simulink model "SimulinkModelEs2"  (R2023a)
settings: Solver=VariableStepAuto  StartTime=0.0  StopTime=100.0  RelTol=1e-3
undefined symbols (not defined in the file or in its folder): fdesignblkfcn, gcbh
libraries: dspfdesign x4, vrlib x1
settings Model: Creator=pisy1  LastModifiedBy=pisy1

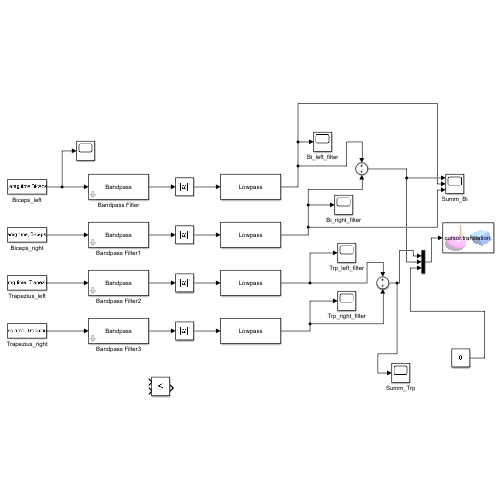
[thumbnail: Simulink's stored preview of the top-level diagram]
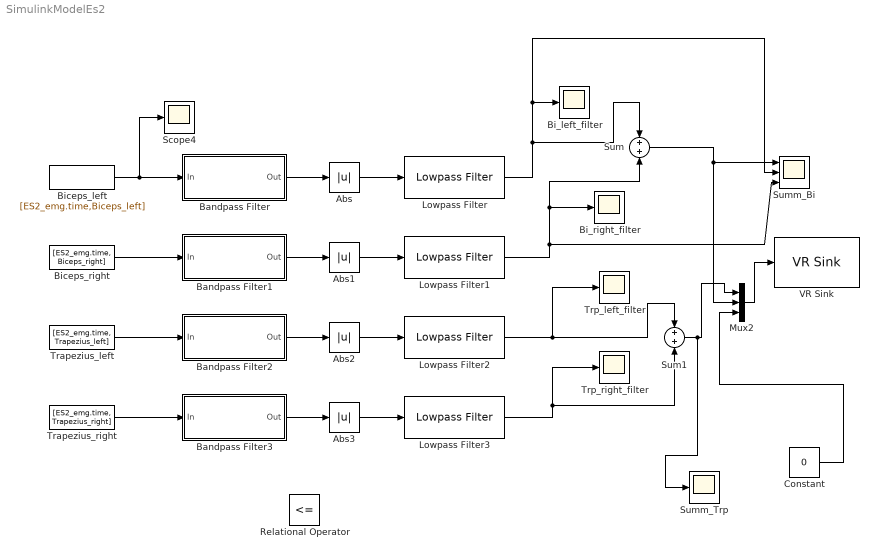
== system SimulinkModelEs2 ==
  Abs{,1..3} (4 alike) : Abs  SaturateOnIntegerOverflow=off
  Bandpass Filter : Subsystem  DialogController=fdesignblkfcn  InitFcn=fdesignblkfcn(gcbh, {'InitFcn'});  mask(Bandpass Filter){}
      mask help: dsp:DSPFilterDesignBlockDialog:BandpassFdesign_MaskDesc
      settings: CopyFcn=fdesignblkfcn(gcbh, {'CopyFcn'});
      mask Help: helpview(mapfilelocation('dsp'), 'dspbandpassfilter');
      mask Display: disp('Bandpass');
  Bandpass Filter1 : Subsystem  DialogController=fdesignblkfcn  InitFcn=fdesignblkfcn(gcbh, {'InitFcn'});  mask(Bandpass Filter){}
      mask help: dsp:DSPFilterDesignBlockDialog:BandpassFdesign_MaskDesc
      settings: CopyFcn=fdesignblkfcn(gcbh, {'CopyFcn'});
      mask Help: helpview(mapfilelocation('dsp'), 'dspbandpassfilter');
      mask Display: disp('Bandpass');
  Bandpass Filter2 : Subsystem  DialogController=fdesignblkfcn  InitFcn=fdesignblkfcn(gcbh, {'InitFcn'});  mask(Bandpass Filter){}
      mask help: dsp:DSPFilterDesignBlockDialog:BandpassFdesign_MaskDesc
      settings: CopyFcn=fdesignblkfcn(gcbh, {'CopyFcn'});
      mask Help: helpview(mapfilelocation('dsp'), 'dspbandpassfilter');
      mask Display: disp('Bandpass');
  Bandpass Filter3 : Subsystem  DialogController=fdesignblkfcn  InitFcn=fdesignblkfcn(gcbh, {'InitFcn'});  mask(Bandpass Filter){}
      mask help: dsp:DSPFilterDesignBlockDialog:BandpassFdesign_MaskDesc
      settings: CopyFcn=fdesignblkfcn(gcbh, {'CopyFcn'});
      mask Help: helpview(mapfilelocation('dsp'), 'dspbandpassfilter');
      mask Display: disp('Bandpass');
  Bi_left_filter : Scope
  Bi_right_filter : Scope
  Biceps_left : FromWorkspace  VariableName=[ES2_emg.time,Biceps_left]  SampleTime=1/1000
  Biceps_right : FromWorkspace  VariableName=[ES2_emg.time, Biceps_right]  SampleTime=1/1000
  Constant : Constant  Value=0
  Lowpass Filter{,1..3} (4 alike) : dspfdesign/Lowpass Filter  FilterType=FIR  DesignForMinimumOrder=on  FilterOrder=50  PassbandFrequency=3  StopbandFrequency=6  PassbandRipple=0.1  StopbandAttenuation=80  SampleRateMode=Specify on dialog  SampleRate=1000  SimulateUsing=Interpreted execution  roundingMode=Floor  coeffsDataTypeStr=fixdt(1,16)
  Mux2 : Mux  Inputs=3
  Relational Operator : RelationalOperator  Operator=<=  OutDataTypeStr=boolean  RndMeth=Simplest  InputSameDT=off
  Scope4 : Scope
  Sum : Sum  Inputs=+|+
  Sum1 : Sum  Inputs=+|+
  Summ_Bi : Scope  NumInputPorts=3
  Summ_Trp : Scope
  "Trapezius_left " : FromWorkspace  VariableName=[ES2_emg.time, Trapezius_left]  SampleTime=1/1000
  Trapezius_right : FromWorkspace  VariableName=[ES2_emg.time, Trapezius_right]  SampleTime=1/1000
  Trp_left_filter : Scope
  Trp_right_filter : Scope
  VR Sink : vrlib/VR Sink  InstantiateOnLoad=on  SampleTime=0.01  ViewEnable=on  RemoteChange=off  RemoteView=off  FieldsWritten=cursor.translation.3.1.1.double  WorldFileName=8_palline_color.wrl  AutoView=off  VideoDimensions=[]  AllowVariableSize=off  FigureProperties="{'Position', 'Name', 'Viewpoint', 'CameraBound', 'CameraDirection', 'CameraPosition', 'CameraUpVector', 'ZoomFactor', 'Antialiasing', 'Headlight', 'Lighting', 'NavPanel', 'Sound', 'StatusBar', 'Stereo3D', 'Stereo3DCameraOffset', 'Stereo3DHIT', 'ToolBar', 'Textures', 'Transparency', 'Triad', 'Wireframe', 'NavZones', 'NavMode', 'NavSpeed', 'CaptureFileFormat', 'CaptureFileName', 'Record2DCompressMethod', 'Record2DCompressQuality', 'Record2D', 'Record2DFileName', 'Record2DFPS'; [5.0000000000000000e+00   9.2000000000000000e+01   5.7600000000000000e+02   3.5000000000000000e+02], '', '_untitled_1', 'on', [0.0000000000000000e+00   0.0000000000000000e+00  -1.0000000000000000e+00], [0.0000000000000000e+00   0.0000000000000000e+00   3.0000000000000000e+00], [0.0000000000000000e+00   1.0000000000000000e+00   0.0000000000000000e+00], [1.0000000000000000e+00], 'on', 'on', 'on', 'halfbar', 'on', 'on', 'off', [1.0000000149011612e-01], [0.0000000000000000e+00], 'on', 'on', 'on', 'none', 'off', 'off', 'fly', 'normal', 'tif', '%f_anim_%n.tif', 'auto', [7.5000000000000000e+01], 'off', '%f_anim_%n.avi', 'auto'}"
  wires:
  Biceps_left/1 -> Scope4/1, Bandpass Filter/1(In)
  Bandpass Filter/1(Out) -> Abs/1
  Abs/1 -> Lowpass Filter/1
  Abs1/1 -> Lowpass Filter1/1
  Bandpass Filter1/1(Out) -> Abs1/1
  Biceps_right/1 -> Bandpass Filter1/1(In)
  Abs2/1 -> Lowpass Filter2/1
  Bandpass Filter2/1(Out) -> Abs2/1
  "Trapezius_left "/1 -> Bandpass Filter2/1(In)
  Trapezius_right/1 -> Bandpass Filter3/1(In)
  Abs3/1 -> Lowpass Filter3/1
  Bandpass Filter3/1(Out) -> Abs3/1
  Lowpass Filter3/1 -> Sum1/2, Trp_right_filter/1
  Lowpass Filter2/1 -> Trp_left_filter/1, Sum1/1
  Lowpass Filter1/1 -> Sum/2, Bi_right_filter/1, Summ_Bi/3
  Constant/1 -> Mux2/3
  Mux2/1 -> VR Sink/1
  Sum1/1 -> Summ_Trp/1, Mux2/1
  Lowpass Filter/1 -> Summ_Bi/2, Bi_left_filter/1, Sum/1
  Sum/1 -> Mux2/2, Summ_Bi/1

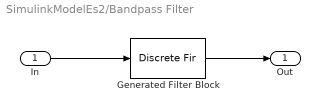
== system SimulinkModelEs2/Bandpass Filter ==
  In : Inport
  Generated Filter Block : DiscreteFir  Tag=BlockMethodSubSystem  Coefficients=[-9.3686702536914806e-06 3.12112809195631884e-05 -4.11531312163778077e-05 3.46959070674858323e-05 -6.95996272654917275e-05 2.25266942632591132e-05 -8.52586640162886797e-05 -1.01275601966525663e-05 -8.19699192663462454e-05 -6.15603887343607549e-05 -5.9928103484218156e-05 -0.000121773920488128754 -2.66693180046293347e-05 -0.000173582148305583721 4.85841196753850187e-06 -0.000196865446555221654 2.09241600116936787e-05 -0.000175070409473414502 1.29594738164580086e-05 -0.00010196560853616344 -1.73899410626521334e-05 1.38497153315267659e-05 -5.64059785452916983e-05 0.000148823711527270122 -8.11137804989736459e-05 0.000269600500847764297 -6.66819945948280264e-05 0.000342503652881703965 3.52069345312515154e-06 0.000344637780110196995 0.00012858070014359381 0.000272834014614537618 0.000285186521797195773 0.000146850926915565155 0.000430093252576786299 4.80147099397023455e-06 0.000510533795609378915 -0.000108659463339479432 0.000480381118947913633 -0.00015808597112364732 0.00031736039761362674 -0.000131661302689836559 3.54013407976428411e-05 -4.87012688565813937e-05 -0.000313041458963056755 4.36426183964740697e-05 -0.00064715606616753366 8.49659330390565632e-05 -0.000878874215356443373 2.38674809802090746e-05 -0.000939300192907026733 -0.000159137006239270498 -0.000802214987435227755 -0.000436425707633868653 -0.000496300153583344693 -0.000732724227282986296 -0.00010054958859877141 -0.00094194330334548609 0.000277523992628194436 -0.000958361368208270319 0.000535344128008414838 -0.000713561015643481011 0.000610103531338323461 -0.000207204782800491044 0.0005029728868787669 0.000479885492686017517 0.000282971816365619878 0.00119743844849929618 6.67763691850669971e-05 0.00176183555280003839 -2.12223470167560569e-05 0.00200788377478970615 0.000103228849646334322 0.00184114661190210136 0.000444622959401494813 0.00127370296145404597 0.000911631333604090194 0.00042976760914902062 0.00133366080069442696 -0.000483818369086393022 0.00150886983424911004 -0.00123599533659225617 0.00127138209007837677 -0.0016422211688103404 0.000557171809006548895 -0.00162513552744896839 -0.000554153422263470546 -0.00124390348382837166 -0.00183920406010100218 -0.000679478097852773263 -0.00297800611694112958 -0.000176737254097106202 -0.0036391164319655952 4.07217243879186256e-05 -0.00357950507876916542 -0.000143667762747536943 -0.0027285210290573284 -0.000682996094840989938 -0.00122710494485526902 -0.00136279543137825189 0.000594984672058177454 -0.00185700203672085201 0.00230266556106554403 -0.00183196437326688718 0.00347853357357814138 -0.00106869689246484384 0.00384924642170408025 0.000436157962248056197 0.00337472332535589245 0.00242774919190852931 0.00226811716984190578 0.00443079990486730003 0.000934428117831991511 0.00586565518688552268 -0.000158568641836894143 0.00621447784239509155 -0.00063968506314412716 0.00518988902168367443 -0.000372975212782562294 0.00285228027553475648 0.000473327518819695217 -0.000367190639521300702 0.00145817426323067989 -0.00375510870797710842 0.00199954564111136943 -0.00649909557305363567 0.00157338850405358815 -0.00791733371223253199 -7.98017159677944681e-05 -0.00766646088654352603 -0.00280949633821852727 -0.00586057658312818218 -0.00602733517521191614 -0.00305626313527977179 -0.00882178250879370185 -9.71425214211978983e-05 -0.0101967846478441017 0.0021442428271443801 -0.0093740351268534923 0.00305308159625901051 -0.00607123588018848061 0.0024971374225030039 -0.000666271859919423284 0.000910364244497557169 0.00581734844136641907 -0.000807046086893129476 0.0119203579027810664 -0.00156048754052804089 0.0161114922324175069 -0.00043720534318062381 0.0172127205975105453 0.00292079817401565914 0.0147655911445284671 0.00806627663117549971 0.0092239105285639323 0.013713884927239137 0.00189815567585120454 0.0179653836624237111 -0.00535739543202795598 0.0187613939058622961 -0.0106502874184987474 0.014459080896858505 -0.0126233469724383804 0.00438953523919432403 -0.0109426370703246453 -0.0107580013276019799 -0.00656125274562321687 ...(+4671 chars)]  InputProcessing=Columns as channels (frame based)
  Out : Outport  VectorParamsAs1DForOutWhenUnconnected=off
  wires:
  In/1 -> Generated Filter Block/1
  Generated Filter Block/1 -> Out/1

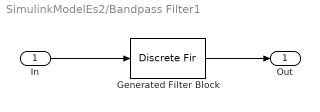
== system SimulinkModelEs2/Bandpass Filter1 ==
  In : Inport
  Generated Filter Block : DiscreteFir  Tag=BlockMethodSubSystem  Coefficients=[-9.3686702536914806e-06 3.12112809195631884e-05 -4.11531312163778077e-05 3.46959070674858323e-05 -6.95996272654917275e-05 2.25266942632591132e-05 -8.52586640162886797e-05 -1.01275601966525663e-05 -8.19699192663462454e-05 -6.15603887343607549e-05 -5.9928103484218156e-05 -0.000121773920488128754 -2.66693180046293347e-05 -0.000173582148305583721 4.85841196753850187e-06 -0.000196865446555221654 2.09241600116936787e-05 -0.000175070409473414502 1.29594738164580086e-05 -0.00010196560853616344 -1.73899410626521334e-05 1.38497153315267659e-05 -5.64059785452916983e-05 0.000148823711527270122 -8.11137804989736459e-05 0.000269600500847764297 -6.66819945948280264e-05 0.000342503652881703965 3.52069345312515154e-06 0.000344637780110196995 0.00012858070014359381 0.000272834014614537618 0.000285186521797195773 0.000146850926915565155 0.000430093252576786299 4.80147099397023455e-06 0.000510533795609378915 -0.000108659463339479432 0.000480381118947913633 -0.00015808597112364732 0.00031736039761362674 -0.000131661302689836559 3.54013407976428411e-05 -4.87012688565813937e-05 -0.000313041458963056755 4.36426183964740697e-05 -0.00064715606616753366 8.49659330390565632e-05 -0.000878874215356443373 2.38674809802090746e-05 -0.000939300192907026733 -0.000159137006239270498 -0.000802214987435227755 -0.000436425707633868653 -0.000496300153583344693 -0.000732724227282986296 -0.00010054958859877141 -0.00094194330334548609 0.000277523992628194436 -0.000958361368208270319 0.000535344128008414838 -0.000713561015643481011 0.000610103531338323461 -0.000207204782800491044 0.0005029728868787669 0.000479885492686017517 0.000282971816365619878 0.00119743844849929618 6.67763691850669971e-05 0.00176183555280003839 -2.12223470167560569e-05 0.00200788377478970615 0.000103228849646334322 0.00184114661190210136 0.000444622959401494813 0.00127370296145404597 0.000911631333604090194 0.00042976760914902062 0.00133366080069442696 -0.000483818369086393022 0.00150886983424911004 -0.00123599533659225617 0.00127138209007837677 -0.0016422211688103404 0.000557171809006548895 -0.00162513552744896839 -0.000554153422263470546 -0.00124390348382837166 -0.00183920406010100218 -0.000679478097852773263 -0.00297800611694112958 -0.000176737254097106202 -0.0036391164319655952 4.07217243879186256e-05 -0.00357950507876916542 -0.000143667762747536943 -0.0027285210290573284 -0.000682996094840989938 -0.00122710494485526902 -0.00136279543137825189 0.000594984672058177454 -0.00185700203672085201 0.00230266556106554403 -0.00183196437326688718 0.00347853357357814138 -0.00106869689246484384 0.00384924642170408025 0.000436157962248056197 0.00337472332535589245 0.00242774919190852931 0.00226811716984190578 0.00443079990486730003 0.000934428117831991511 0.00586565518688552268 -0.000158568641836894143 0.00621447784239509155 -0.00063968506314412716 0.00518988902168367443 -0.000372975212782562294 0.00285228027553475648 0.000473327518819695217 -0.000367190639521300702 0.00145817426323067989 -0.00375510870797710842 0.00199954564111136943 -0.00649909557305363567 0.00157338850405358815 -0.00791733371223253199 -7.98017159677944681e-05 -0.00766646088654352603 -0.00280949633821852727 -0.00586057658312818218 -0.00602733517521191614 -0.00305626313527977179 -0.00882178250879370185 -9.71425214211978983e-05 -0.0101967846478441017 0.0021442428271443801 -0.0093740351268534923 0.00305308159625901051 -0.00607123588018848061 0.0024971374225030039 -0.000666271859919423284 0.000910364244497557169 0.00581734844136641907 -0.000807046086893129476 0.0119203579027810664 -0.00156048754052804089 0.0161114922324175069 -0.00043720534318062381 0.0172127205975105453 0.00292079817401565914 0.0147655911445284671 0.00806627663117549971 0.0092239105285639323 0.013713884927239137 0.00189815567585120454 0.0179653836624237111 -0.00535739543202795598 0.0187613939058622961 -0.0106502874184987474 0.014459080896858505 -0.0126233469724383804 0.00438953523919432403 -0.0109426370703246453 -0.0107580013276019799 -0.00656125274562321687 ...(+4671 chars)]  InputProcessing=Columns as channels (frame based)
  Out : Outport  VectorParamsAs1DForOutWhenUnconnected=off
  wires:
  In/1 -> Generated Filter Block/1
  Generated Filter Block/1 -> Out/1

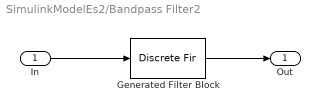
== system SimulinkModelEs2/Bandpass Filter2 ==
  In : Inport
  Generated Filter Block : DiscreteFir  Tag=BlockMethodSubSystem  Coefficients=[-9.3686702536914806e-06 3.12112809195631884e-05 -4.11531312163778077e-05 3.46959070674858323e-05 -6.95996272654917275e-05 2.25266942632591132e-05 -8.52586640162886797e-05 -1.01275601966525663e-05 -8.19699192663462454e-05 -6.15603887343607549e-05 -5.9928103484218156e-05 -0.000121773920488128754 -2.66693180046293347e-05 -0.000173582148305583721 4.85841196753850187e-06 -0.000196865446555221654 2.09241600116936787e-05 -0.000175070409473414502 1.29594738164580086e-05 -0.00010196560853616344 -1.73899410626521334e-05 1.38497153315267659e-05 -5.64059785452916983e-05 0.000148823711527270122 -8.11137804989736459e-05 0.000269600500847764297 -6.66819945948280264e-05 0.000342503652881703965 3.52069345312515154e-06 0.000344637780110196995 0.00012858070014359381 0.000272834014614537618 0.000285186521797195773 0.000146850926915565155 0.000430093252576786299 4.80147099397023455e-06 0.000510533795609378915 -0.000108659463339479432 0.000480381118947913633 -0.00015808597112364732 0.00031736039761362674 -0.000131661302689836559 3.54013407976428411e-05 -4.87012688565813937e-05 -0.000313041458963056755 4.36426183964740697e-05 -0.00064715606616753366 8.49659330390565632e-05 -0.000878874215356443373 2.38674809802090746e-05 -0.000939300192907026733 -0.000159137006239270498 -0.000802214987435227755 -0.000436425707633868653 -0.000496300153583344693 -0.000732724227282986296 -0.00010054958859877141 -0.00094194330334548609 0.000277523992628194436 -0.000958361368208270319 0.000535344128008414838 -0.000713561015643481011 0.000610103531338323461 -0.000207204782800491044 0.0005029728868787669 0.000479885492686017517 0.000282971816365619878 0.00119743844849929618 6.67763691850669971e-05 0.00176183555280003839 -2.12223470167560569e-05 0.00200788377478970615 0.000103228849646334322 0.00184114661190210136 0.000444622959401494813 0.00127370296145404597 0.000911631333604090194 0.00042976760914902062 0.00133366080069442696 -0.000483818369086393022 0.00150886983424911004 -0.00123599533659225617 0.00127138209007837677 -0.0016422211688103404 0.000557171809006548895 -0.00162513552744896839 -0.000554153422263470546 -0.00124390348382837166 -0.00183920406010100218 -0.000679478097852773263 -0.00297800611694112958 -0.000176737254097106202 -0.0036391164319655952 4.07217243879186256e-05 -0.00357950507876916542 -0.000143667762747536943 -0.0027285210290573284 -0.000682996094840989938 -0.00122710494485526902 -0.00136279543137825189 0.000594984672058177454 -0.00185700203672085201 0.00230266556106554403 -0.00183196437326688718 0.00347853357357814138 -0.00106869689246484384 0.00384924642170408025 0.000436157962248056197 0.00337472332535589245 0.00242774919190852931 0.00226811716984190578 0.00443079990486730003 0.000934428117831991511 0.00586565518688552268 -0.000158568641836894143 0.00621447784239509155 -0.00063968506314412716 0.00518988902168367443 -0.000372975212782562294 0.00285228027553475648 0.000473327518819695217 -0.000367190639521300702 0.00145817426323067989 -0.00375510870797710842 0.00199954564111136943 -0.00649909557305363567 0.00157338850405358815 -0.00791733371223253199 -7.98017159677944681e-05 -0.00766646088654352603 -0.00280949633821852727 -0.00586057658312818218 -0.00602733517521191614 -0.00305626313527977179 -0.00882178250879370185 -9.71425214211978983e-05 -0.0101967846478441017 0.0021442428271443801 -0.0093740351268534923 0.00305308159625901051 -0.00607123588018848061 0.0024971374225030039 -0.000666271859919423284 0.000910364244497557169 0.00581734844136641907 -0.000807046086893129476 0.0119203579027810664 -0.00156048754052804089 0.0161114922324175069 -0.00043720534318062381 0.0172127205975105453 0.00292079817401565914 0.0147655911445284671 0.00806627663117549971 0.0092239105285639323 0.013713884927239137 0.00189815567585120454 0.0179653836624237111 -0.00535739543202795598 0.0187613939058622961 -0.0106502874184987474 0.014459080896858505 -0.0126233469724383804 0.00438953523919432403 -0.0109426370703246453 -0.0107580013276019799 -0.00656125274562321687 ...(+4671 chars)]  InputProcessing=Columns as channels (frame based)
  Out : Outport  VectorParamsAs1DForOutWhenUnconnected=off
  wires:
  In/1 -> Generated Filter Block/1
  Generated Filter Block/1 -> Out/1

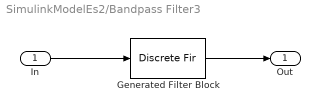
== system SimulinkModelEs2/Bandpass Filter3 ==
  In : Inport
  Generated Filter Block : DiscreteFir  Tag=BlockMethodSubSystem  Coefficients=[-9.3686702536914806e-06 3.12112809195631884e-05 -4.11531312163778077e-05 3.46959070674858323e-05 -6.95996272654917275e-05 2.25266942632591132e-05 -8.52586640162886797e-05 -1.01275601966525663e-05 -8.19699192663462454e-05 -6.15603887343607549e-05 -5.9928103484218156e-05 -0.000121773920488128754 -2.66693180046293347e-05 -0.000173582148305583721 4.85841196753850187e-06 -0.000196865446555221654 2.09241600116936787e-05 -0.000175070409473414502 1.29594738164580086e-05 -0.00010196560853616344 -1.73899410626521334e-05 1.38497153315267659e-05 -5.64059785452916983e-05 0.000148823711527270122 -8.11137804989736459e-05 0.000269600500847764297 -6.66819945948280264e-05 0.000342503652881703965 3.52069345312515154e-06 0.000344637780110196995 0.00012858070014359381 0.000272834014614537618 0.000285186521797195773 0.000146850926915565155 0.000430093252576786299 4.80147099397023455e-06 0.000510533795609378915 -0.000108659463339479432 0.000480381118947913633 -0.00015808597112364732 0.00031736039761362674 -0.000131661302689836559 3.54013407976428411e-05 -4.87012688565813937e-05 -0.000313041458963056755 4.36426183964740697e-05 -0.00064715606616753366 8.49659330390565632e-05 -0.000878874215356443373 2.38674809802090746e-05 -0.000939300192907026733 -0.000159137006239270498 -0.000802214987435227755 -0.000436425707633868653 -0.000496300153583344693 -0.000732724227282986296 -0.00010054958859877141 -0.00094194330334548609 0.000277523992628194436 -0.000958361368208270319 0.000535344128008414838 -0.000713561015643481011 0.000610103531338323461 -0.000207204782800491044 0.0005029728868787669 0.000479885492686017517 0.000282971816365619878 0.00119743844849929618 6.67763691850669971e-05 0.00176183555280003839 -2.12223470167560569e-05 0.00200788377478970615 0.000103228849646334322 0.00184114661190210136 0.000444622959401494813 0.00127370296145404597 0.000911631333604090194 0.00042976760914902062 0.00133366080069442696 -0.000483818369086393022 0.00150886983424911004 -0.00123599533659225617 0.00127138209007837677 -0.0016422211688103404 0.000557171809006548895 -0.00162513552744896839 -0.000554153422263470546 -0.00124390348382837166 -0.00183920406010100218 -0.000679478097852773263 -0.00297800611694112958 -0.000176737254097106202 -0.0036391164319655952 4.07217243879186256e-05 -0.00357950507876916542 -0.000143667762747536943 -0.0027285210290573284 -0.000682996094840989938 -0.00122710494485526902 -0.00136279543137825189 0.000594984672058177454 -0.00185700203672085201 0.00230266556106554403 -0.00183196437326688718 0.00347853357357814138 -0.00106869689246484384 0.00384924642170408025 0.000436157962248056197 0.00337472332535589245 0.00242774919190852931 0.00226811716984190578 0.00443079990486730003 0.000934428117831991511 0.00586565518688552268 -0.000158568641836894143 0.00621447784239509155 -0.00063968506314412716 0.00518988902168367443 -0.000372975212782562294 0.00285228027553475648 0.000473327518819695217 -0.000367190639521300702 0.00145817426323067989 -0.00375510870797710842 0.00199954564111136943 -0.00649909557305363567 0.00157338850405358815 -0.00791733371223253199 -7.98017159677944681e-05 -0.00766646088654352603 -0.00280949633821852727 -0.00586057658312818218 -0.00602733517521191614 -0.00305626313527977179 -0.00882178250879370185 -9.71425214211978983e-05 -0.0101967846478441017 0.0021442428271443801 -0.0093740351268534923 0.00305308159625901051 -0.00607123588018848061 0.0024971374225030039 -0.000666271859919423284 0.000910364244497557169 0.00581734844136641907 -0.000807046086893129476 0.0119203579027810664 -0.00156048754052804089 0.0161114922324175069 -0.00043720534318062381 0.0172127205975105453 0.00292079817401565914 0.0147655911445284671 0.00806627663117549971 0.0092239105285639323 0.013713884927239137 0.00189815567585120454 0.0179653836624237111 -0.00535739543202795598 0.0187613939058622961 -0.0106502874184987474 0.014459080896858505 -0.0126233469724383804 0.00438953523919432403 -0.0109426370703246453 -0.0107580013276019799 -0.00656125274562321687 ...(+4671 chars)]  InputProcessing=Columns as channels (frame based)
  Out : Outport  VectorParamsAs1DForOutWhenUnconnected=off
  wires:
  In/1 -> Generated Filter Block/1
  Generated Filter Block/1 -> Out/1
